simulink model "groundStation001_th"  (R2018b)
settings: Solver=VariableStepAuto  StartTime=0.0  StopTime=sim_time  FixedStep=1e-2  MaxStep=.1  RelTol=1e-3
values from neighbouring files (symbols this model uses):
  wnch = OCT.winches    [groundStation001_ts.m]
libraries: groundStation001_cl x1, waveFlow_ul x1
settings Model: SimulationMode=accelerator  Creator=Erin B  LastModifiedBy=mcobb

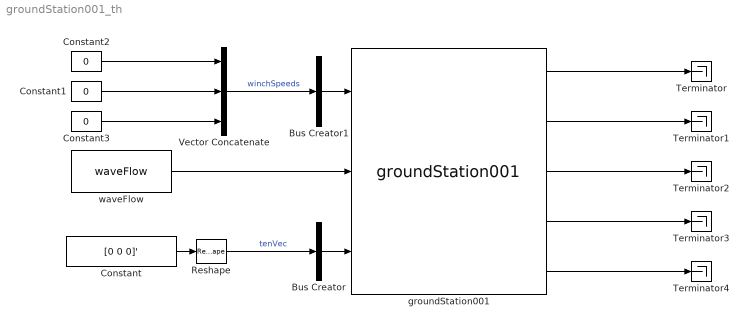
== system groundStation001_th ==
  Bus Creator : BusCreator  Inputs=1  OutDataTypeStr=Bus: thrTenVecBus  NonVirtualBus=on
  Bus Creator1 : BusCreator  Inputs=1  OutDataTypeStr=Bus: gndStnCtrlBus  NonVirtualBus=on
  Constant : Constant  Value=[0 0 0]'
  Constant1 : Constant  Value=0
  Constant2 : Constant  Value=0
  Constant3 : Constant  Value=0
  Reshape : Reshape  OutputDimensionality=Column vector (2-D)
  Terminator{,1..4} (5 alike) : Terminator
  Vector Concatenate : Concatenate  NumInputs=3
  groundStation001 : groundStation001_cl/groundStation001  gs=gndStn  e=env  numNodes=gndStn.anchThrs.numNodes.Value  anchWnchStruct=wnch.struct('OCT.winch')
  waveFlow : waveFlow_ul/waveFlow  e=env.water
  wires:
  groundStation001/1 -> Terminator/1
  Bus Creator/1 -> groundStation001/3
  Reshape/1 -> Bus Creator/1  "tenVec"
  Bus Creator1/1 -> groundStation001/1
  waveFlow/1 -> groundStation001/2
  Vector Concatenate/1 -> Bus Creator1/1  "winchSpeeds"
  Constant1/1 -> Vector Concatenate/2
  Constant2/1 -> Vector Concatenate/1
  Constant3/1 -> Vector Concatenate/3
  Constant/1 -> Reshape/1
  groundStation001/2 -> Terminator1/1
  groundStation001/3 -> Terminator2/1
  groundStation001/4 -> Terminator3/1
  groundStation001/5 -> Terminator4/1
